simulink model "Pressure_Drop_Collector_example"  (Simulink 7.6)
settings: Solver=ode45  StartTime=0.0  StopTime=10.0  RelTol=1e-3
libraries: carnot x3
settings Model: Creator=drhf  LastModifiedBy=drhf

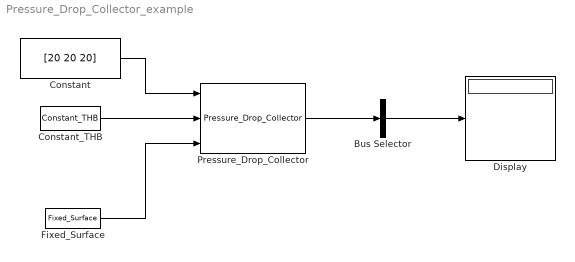
== system Pressure_Drop_Collector_example ==
  Bus Selector : BusSelector  OutputSignals=Pressure,GeodeticHeight  OutputAsBus=on
  Constant : Constant  Value=[20 20 20]
  Constant_THB : carnot/Source/Simple/Constant_THB  SystemSampleTime=-1  t=40  mdot=200/3600  p=2e5  mID=Full Pressure Drop with Static Height  fluid=water  mix=0  dia=0.02  hgt=10
  Display : Display
  Fixed_Surface : carnot/Weather/Fixed_Surface  SystemSampleTime=-1  colangle=30  colazi=0  colrot=0
  Pressure_Drop_Collector : carnot/Basic/Pressure_Drop/Pressure_Drop_Collector  SystemSampleTime=-1  len=1  lin=10  qua=10
  wires:
  Constant_THB/1 -> Pressure_Drop_Collector/2
  Constant/1 -> Pressure_Drop_Collector/1
  Pressure_Drop_Collector/1 -> Bus Selector/1
  Bus Selector/1 -> Display/1
  Fixed_Surface/1 -> Pressure_Drop_Collector/3
